simulink model "vibration2"  (R2022b)
settings: Solver=VariableStepAuto  StartTime=0.0  StopTime=10.0  RelTol=1e-3
undefined symbols (not defined in the file or in its folder): magnitude
settings Model: Creator=integzz  LastModifiedBy=integzz

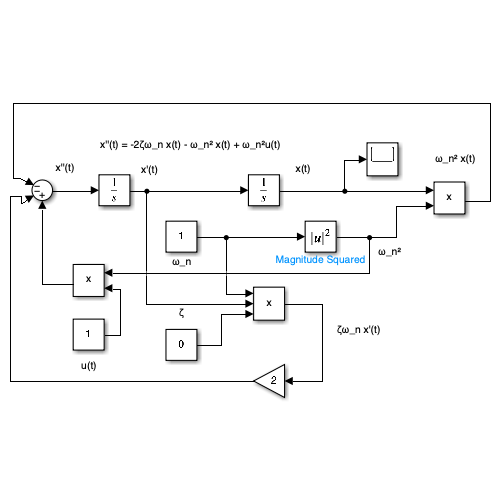
[thumbnail: Simulink's stored preview of the top-level diagram]
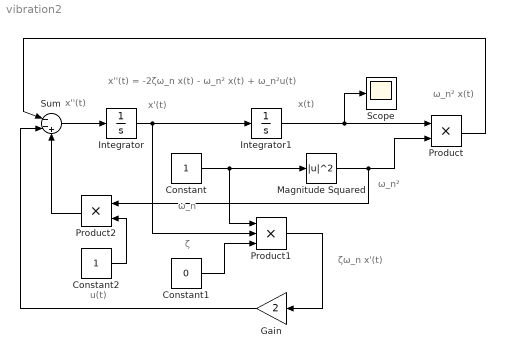
== system vibration2 ==
  note: ζ
  note: ω_n
  note: ζω_n x'(t)
  note: ω_n² x(t)
  note: x''(t)
  note: x''(t) = -2ζω_n x(t) - ω_n² x(t) + ω_n²u(t)
  note: x'(t)
  note: x(t)
  note: u(t)
  note: ω_n²
  Constant : Constant
  Constant1 : Constant  Value=0
  Constant2 : Constant
  Gain : Gain  Gain=2
  Integrator : Integrator
  Integrator1 : Integrator  InitialCondition=5
  Magnitude Squared : Math  Operator=magnitude^2
  Product : Product
  Product1 : Product  Inputs=3
  Product2 : Product
  Scope : Scope
  Sum : Sum  Inputs=|--+
  wires:
  Magnitude Squared/1 -> Product2/1, Product/2
  Product/1 -> Sum/1
  Integrator/1 -> Product1/2, Integrator1/1
  Gain/1 -> Sum/2
  Constant/1 -> Magnitude Squared/1, Product1/1
  Integrator1/1 -> Scope/1, Product/1
  Sum/1 -> Integrator/1
  Constant1/1 -> Product1/3
  Product1/1 -> Gain/1
  Product2/1 -> Sum/3
  Constant2/1 -> Product2/2
